simulink model "sei"  (Simulink 6.2)
settings: Solver=ode45  StartTime=0.0  StopTime=10.0  RelTol=1e-3
libraries: dsparch4 x287, cdsEpicsOut x108, cdsEpicsIn x18, cdsRms x18, Matrix8x x15, cdsSwitch1 x12, cdsProduct x9, Matrix88 x9, cdsSwitch x6, cdsSubtract8 x3, cdsRampSwitch x3, cdsSWD1 x3
(part 1 of 6)
settings Model: LastModifiedBy=rolf
settings DebuggingCC: SolverPrmCheckMsg=warning

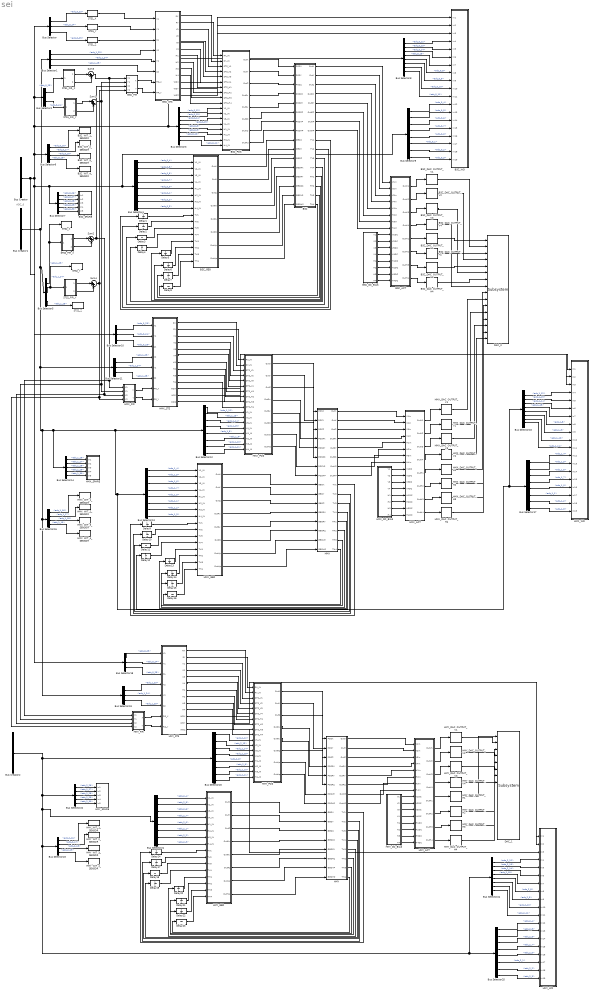
== system sei ==
  note: ADC_0
  BSC : Subsystem
  BSC_ACT : Subsystem
  BSC_DAC_OUTPUT_H{1..4} (4 alike) : cdsEpicsOut/Subsystem
  BSC_DAC_OUTPUT_V{1..4} (4 alike) : cdsEpicsOut/Subsystem
  BSC_DC_BIAS : Subsystem
  BSC_FIR : Subsystem
  BSC_GEO : Subsystem
  BSC_POS : Subsystem
  BSC_SPARE : Subsystem
  BSC_STS : Subsystem
  BSC_WD : Subsystem
  BSC_WIT_1_SENSOR : cdsEpicsOut/Subsystem
  BSC_WIT_2_SENSOR : cdsEpicsOut/Subsystem
  BSC_WIT_3_SENSOR : cdsEpicsOut/Subsystem
  BSC_WIT_4_SENSOR : cdsEpicsOut/Subsystem
  Bus Creator : BusCreator  Inputs='adc_0_0','adc_0_1','adc_0_2','adc_0_3','adc_0_4','adc_0_5','adc_0_6','adc_0_7','adc_0_8','adc_0_9','adc_0_10','adc_0_11','adc_0_12','adc_0_13','adc_0_14','adc_0_15','adc_0_16','adc_0_17','adc_0_18','adc_0_19','adc_0_20','adc_0_21','adc_0_22','adc_0_23','adc_0_24','adc_0_25','adc_0_26','adc_0_27','adc_0_28','adc_0_29','adc_0_30','adc_0_31'
  Bus Creator1 : BusCreator  Inputs='adc_1_0','adc_1_1','adc_1_2','adc_1_3','adc_1_4','adc_1_5','adc_1_6','adc_1_7','adc_1_8','adc_1_9','adc_1_10','adc_1_11','adc_1_12','adc_1_13','adc_1_14','adc_1_15','adc_1_16','adc_1_17','adc_1_18','adc_1_19','adc_1_20','adc_1_21','adc_1_22','adc_1_23','adc_1_24','adc_1_25','adc_1_26','adc_1_27','adc_1_28','adc_1_29','adc_1_30','adc_1_31'
  Bus Creator2 : BusCreator  Inputs='adc_2_0','adc_2_1','adc_2_2','adc_2_3','adc_2_4','adc_2_5','adc_2_6','adc_2_7','adc_2_8','adc_2_9','adc_2_10','adc_2_11','adc_2_12','adc_2_13','adc_2_14','adc_2_15','adc_2_16','adc_2_17','adc_2_18','adc_2_19','adc_2_20','adc_2_21','adc_2_22','adc_2_23','adc_2_24','adc_2_25','adc_2_26','adc_2_27','adc_2_28','adc_2_29','adc_2_30','adc_2_31'
  Bus Selector : BusSelector  OutputSignals=adc_0_23,adc_0_24,adc_0_25
  Bus Selector{1,5,11,19} (4 alike) : BusSelector  OutputSignals=adc_1_23,adc_1_24,adc_1_25
  Bus Selector10 : BusSelector  OutputSignals=adc_0_23,adc_0_24,adc_0_25
  Bus Selector12 : BusSelector  OutputSignals=adc_1_12,adc_1_13,adc_1_14,adc_1_15,adc_1_8,adc_1_9,adc_1_10,adc_1_11
  Bus Selector13 : BusSelector  OutputSignals=adc_1_4,adc_1_5,adc_1_6,adc_1_7,adc_1_0,adc_1_1,adc_1_2,adc_1_3
  Bus Selector14 : BusSelector  OutputSignals=adc_1_26,adc_1_27,adc_1_28,adc_1_29,adc_1_30
  Bus Selector15 : BusSelector  OutputSignals=adc_1_16,adc_1_17,adc_1_18,adc_1_19
  Bus Selector16 : BusSelector  OutputSignals=adc_1_12,adc_1_13,adc_1_14,adc_1_15,adc_1_8,adc_1_9,adc_1_10,adc_1_11
  Bus Selector17 : BusSelector  OutputSignals=adc_1_4,adc_1_5,adc_1_6,adc_1_7,adc_1_0,adc_1_1,adc_1_2,adc_1_3
  Bus Selector18 : BusSelector  OutputSignals=adc_0_23,adc_0_24,adc_0_25
  Bus Selector2 : BusSelector  OutputSignals=adc_0_23,adc_0_24
  Bus Selector20 : BusSelector  OutputSignals=adc_2_12,adc_2_13,adc_2_14,adc_2_15,adc_2_8,adc_2_9,adc_2_10,adc_2_11
  Bus Selector21 : BusSelector  OutputSignals=adc_2_4,adc_2_5,adc_2_6,adc_2_7,adc_2_0,adc_2_1,adc_2_2,adc_2_3
  Bus Selector22 : BusSelector  OutputSignals=adc_2_26,adc_2_27,adc_2_28,adc_2_29,adc_2_30
  Bus Selector23 : BusSelector  OutputSignals=adc_2_16,adc_2_17,adc_2_18,adc_2_19
  Bus Selector24 : BusSelector  OutputSignals=adc_2_12,adc_2_13,adc_2_14,adc_2_15,adc_2_8,adc_2_9,adc_2_10,adc_2_11
  Bus Selector25 : BusSelector  OutputSignals=adc_2_4,adc_2_5,adc_2_6,adc_2_7,adc_2_0,adc_2_1,adc_2_2,adc_2_3
  Bus Selector3 : BusSelector  OutputSignals=adc_0_12,adc_0_13,adc_0_14,adc_0_15,adc_0_8,adc_0_9,adc_0_10,adc_0_11
  Bus Selector4 : BusSelector  OutputSignals=adc_0_4,adc_0_5,adc_0_6,adc_0_7,adc_0_0,adc_0_1,adc_0_2,adc_0_3
  Bus Selector6 : BusSelector  OutputSignals=adc_0_16,adc_0_17,adc_0_18,adc_0_19
  Bus Selector7 : BusSelector  OutputSignals=adc_0_26,adc_0_27,adc_0_28,adc_0_29,adc_0_30
  Bus Selector8 : BusSelector  OutputSignals=adc_0_12,adc_0_13,adc_0_14,adc_0_15,adc_0_8,adc_0_9,adc_0_10,adc_0_11
  Bus Selector9 : BusSelector  OutputSignals=adc_0_4,adc_0_5,adc_0_6,adc_0_7,adc_0_0,adc_0_1,adc_0_2,adc_0_3
  DAC_0 : dac/Subsystem
  DAC_1 : dac/Subsystem
  Delay{1..24} (24 alike) : UnitDelay
  HMX : Subsystem
  HMX_ACT : Subsystem
  HMX_DAC_OUTPUT_H{1..4} (4 alike) : cdsEpicsOut/Subsystem
  HMX_DAC_OUTPUT_V{1..4} (4 alike) : cdsEpicsOut/Subsystem
  HMX_DC_BIAS : Subsystem
  HMX_FIR : Subsystem
  HMX_GEO : Subsystem
  HMX_POS : Subsystem
  HMX_SPARE : Subsystem
  HMX_STS : Subsystem
  HMX_WD : Subsystem
  HMX_WIT_1_SENSOR : cdsEpicsOut/Subsystem
  HMX_WIT_2_SENSOR : cdsEpicsOut/Subsystem
  HMX_WIT_3_SENSOR : cdsEpicsOut/Subsystem
  HMX_WIT_4_SENSOR : cdsEpicsOut/Subsystem
  HMY : Subsystem
  HMY_ACT : Subsystem
  HMY_DAC_OUTPUT_H{1..4} (4 alike) : cdsEpicsOut/Subsystem
  HMY_DAC_OUTPUT_V{1..4} (4 alike) : cdsEpicsOut/Subsystem
  HMY_DC_BIAS : Subsystem
  HMY_FIR : Subsystem
  HMY_GEO : Subsystem
  HMY_POS : Subsystem
  HMY_SPARE : Subsystem
  HMY_STS : Subsystem
  HMY_WD : Subsystem
  HMY_WIT_1_SENSOR : cdsEpicsOut/Subsystem
  HMY_WIT_2_SENSOR : cdsEpicsOut/Subsystem
  HMY_WIT_3_SENSOR : cdsEpicsOut/Subsystem
  HMY_WIT_4_SENSOR : cdsEpicsOut/Subsystem
  STS1_FIR_X : Subsystem
  STS1_FIR_Y : Subsystem
  STS1_X : cdsEpicsOut/Subsystem
  STS1_Y : cdsEpicsOut/Subsystem
  STS1_Z : cdsEpicsOut/Subsystem
  STS2_FIR_X : Subsystem
  STS2_FIR_Y : Subsystem
  STS2_X : cdsEpicsOut/Subsystem
  STS2_Y : cdsEpicsOut/Subsystem
  STS2_Z : cdsEpicsOut/Subsystem
  Sum{1..4} (4 alike) : Sum  Inputs=|++
  wires:
  BSC_FIR/1(X) -> BSC_STS/7(FIR_X)
  BSC_FIR/2(Y) -> BSC_STS/8(FIR_Y)
  BSC/1(OutX) -> BSC_ACT/1(V1In)
  BSC/2(OutY) -> BSC_ACT/2(V2In)
  BSC/3(OutZ) -> BSC_ACT/3(V3In)
  BSC/4(OutRX) -> BSC_ACT/4(V4In)
  BSC/5(OutRY) -> BSC_ACT/5(H1In)
  BSC/6(OutRZ) -> BSC_ACT/6(H2In)
  BSC/7(OutVP) -> BSC_ACT/7(H3In)
  BSC/8(OutHP) -> BSC_ACT/8(H4In)
  BSC_STS/10(H4) -> BSC_POS/10(STS_H4)
  BSC_STS/9(H3) -> BSC_POS/9(STS_H3)
  BSC_STS/8(H2) -> BSC_POS/8(STS_H2)
  BSC_STS/7(H1) -> BSC_POS/7(STS_H1)
  BSC_STS/6(V4) -> BSC_POS/6(STS_V4)
  BSC_STS/5(V3) -> BSC_POS/5(STS_V3)
  BSC_STS/4(V2) -> BSC_POS/4(STS_V2)
  BSC_STS/3(V1) -> BSC_POS/3(STS_V1)
  BSC_POS/1(OutX) -> BSC/1(POSX)
  BSC_POS/2(OutY) -> BSC/2(POSY)
  BSC_POS/3(OutZ) -> BSC/3(POSZ)
  BSC_POS/4(OutRx) -> BSC/4(POSRX)
  BSC_POS/5(OutRy) -> BSC/5(POSRY)
  BSC_POS/6(OutRZ) -> BSC/6(POSRZ)
  BSC_POS/7(OutVp) -> BSC/7(POSVP)
  BSC_POS/8(OutHp) -> BSC/8(POSHP)
  BSC_GEO/1(OutX) -> BSC/9(GEOX)
  BSC_GEO/2(OutY) -> BSC/10(GEOY)
  BSC_GEO/3(OutZ) -> BSC/11(GEOZ)
  BSC_GEO/4(OutRx) -> BSC/12(GEORX)
  BSC_GEO/5(OutRy) -> BSC/13(GEORY)
  BSC_GEO/6(OutRz) -> BSC/14(GEORZ)
  BSC_GEO/7(OutVp) -> BSC/15(GEOVP)
  BSC_GEO/8(OutHp) -> BSC/16(GEOHP)
  Bus Creator/1 -> Bus Selector/1, Bus Selector2/1, Bus Selector3/1, Bus Selector8/1, Bus Selector6/1, Bus Selector7/1, Bus Selector4/1, Bus Selector9/1, Bus Selector10/1, Bus Selector18/1
  Bus Creator1/1 -> Bus Selector1/1, Bus Selector5/1, Bus Selector11/1, Bus Selector12/1, Bus Selector13/1, Bus Selector17/1, Bus Selector16/1, Bus Selector14/1, Bus Selector15/1, Bus Selector19/1
  Bus Selector1/1 -> BSC_STS/4(X2)  "<adc_1_23>"
  Bus Selector1/2 -> BSC_STS/5(Y2)  "<adc_1_24>"
  Bus Selector1/3 -> BSC_STS/6(Z2)  "<adc_1_25>"
  Bus Selector3/1 -> BSC_POS/11(V1_IN)  "<adc_0_12>"
  Bus Selector3/2 -> BSC_POS/12(V2_IN)  "<adc_0_13>"
  Bus Selector3/3 -> BSC_POS/13(V3_IN)  "<adc_0_14>"
  Bus Selector3/4 -> BSC_POS/14(V4_IN)  "<adc_0_15>"
  Bus Selector3/5 -> BSC_POS/15(H1_IN)  "<adc_0_8>"
  Bus Selector3/6 -> BSC_POS/16(H2_IN)  "<adc_0_9>"
  Bus Selector3/7 -> BSC_POS/17(H3_IN)  "<adc_0_10>"
  Bus Selector3/8 -> BSC_POS/18(H4_IN)  "<adc_0_11>"
  Bus Selector/1 -> STS1_X/1  "<adc_0_23>"
  Bus Selector/2 -> STS1_Y/1  "<adc_0_24>"
  Bus Selector/3 -> STS1_Z/1  "<adc_0_25>"
  STS1_X/1 -> BSC_STS/1(X1)
  STS1_Y/1 -> BSC_STS/2(Y1)
  STS1_Z/1 -> BSC_STS/3(Z1)
  BSC_ACT/1(OutV1) -> BSC_DAC_OUTPUT_V1/1
  BSC_ACT/2(OutV2) -> BSC_DAC_OUTPUT_V2/1
  BSC_ACT/3(OutV3) -> BSC_DAC_OUTPUT_V3/1
  BSC_ACT/4(OutV4) -> BSC_DAC_OUTPUT_V4/1
  BSC_ACT/5(OutH1) -> BSC_DAC_OUTPUT_H1/1
  BSC_ACT/6(OutH2) -> BSC_DAC_OUTPUT_H2/1
  BSC_ACT/7(OutH3) -> BSC_DAC_OUTPUT_H3/1
  BSC_ACT/8(OutH4) -> BSC_DAC_OUTPUT_H4/1
  BSC_DC_BIAS/1(V1) -> BSC_ACT/9(V1DC)
  BSC_DC_BIAS/2(V2) -> BSC_ACT/10(V2DC)
  BSC_DC_BIAS/3(V3) -> BSC_ACT/11(V3DC)
  BSC_DC_BIAS/4(V4) -> BSC_ACT/12(V4DC)
  BSC_DC_BIAS/5(H1) -> BSC_ACT/13(H1DC)
  BSC_DC_BIAS/6(H2) -> BSC_ACT/14(H2DC)
  BSC_DC_BIAS/7(H3) -> BSC_ACT/15(H3DC)
  BSC_DC_BIAS/8(H4) -> BSC_ACT/16(H4DC)
  Delay1/1 -> BSC_GEO/9(TV1)
  Delay2/1 -> BSC_GEO/10(TV2)
  Delay8/1 -> BSC_GEO/16(TH4)
  Delay7/1 -> BSC_GEO/15(TH3)
  Delay6/1 -> BSC_GEO/14(TH2)
  Delay5/1 -> BSC_GEO/13(TH1)
  BSC/16(TH4) -> Delay8/1
  BSC/15(TH3) -> Delay7/1
  BSC/14(TH2) -> Delay6/1
  BSC/13(TH1) -> Delay5/1
  Delay3/1 -> BSC_GEO/11(TV3)
  Delay4/1 -> BSC_GEO/12(TV4)
  BSC/12(TV4) -> Delay4/1
  BSC/11(TV3) -> Delay3/1
  BSC/10(TV2) -> Delay2/1
  BSC/9(TV1) -> Delay1/1
  BSC_DAC_OUTPUT_H1/1 -> DAC_0/1
  BSC_DAC_OUTPUT_V1/1 -> DAC_0/2
  BSC_DAC_OUTPUT_H2/1 -> DAC_0/3
  BSC_DAC_OUTPUT_V2/1 -> DAC_0/4
  BSC_DAC_OUTPUT_H3/1 -> DAC_0/5
  BSC_DAC_OUTPUT_V3/1 -> DAC_0/6
  BSC_DAC_OUTPUT_V4/1 -> DAC_0/8
  Bus Selector6/1 -> BSC_WIT_1_SENSOR/1  "<adc_0_16>"
  Bus Selector6/2 -> BSC_WIT_2_SENSOR/1  "<adc_0_17>"
  Bus Selector6/3 -> BSC_WIT_3_SENSOR/1  "<adc_0_18>"
  Bus Selector6/4 -> BSC_WIT_4_SENSOR/1  "<adc_0_19>"
  Bus Selector7/1 -> BSC_SPARE/1(In1)  "<adc_0_26>"
  Bus Selector7/2 -> BSC_SPARE/2(In2)  "<adc_0_27>"
  Bus Selector7/3 -> BSC_SPARE/3(In3)  "<adc_0_28>"
  Bus Selector7/4 -> BSC_SPARE/4(In4)  "<adc_0_29>"
  Bus Selector7/5 -> BSC_SPARE/5(In5)  "<adc_0_30>"
  Bus Selector4/8 -> BSC_GEO/8(H4_IN)  "<adc_0_3>"
  Bus Selector4/7 -> BSC_GEO/7(H3_IN)  "<adc_0_2>"
  Bus Selector4/6 -> BSC_GEO/6(H2_IN)  "<adc_0_1>"
  Bus Selector4/5 -> BSC_GEO/5(H1_IN)  "<adc_0_0>"
  Bus Selector4/4 -> BSC_GEO/4(V4_IN)  "<adc_0_7>"
  Bus Selector4/3 -> BSC_GEO/3(V3_IN)  "<adc_0_6>"
  Bus Selector4/2 -> BSC_GEO/2(V2_IN)  "<adc_0_5>"
  Bus Selector4/1 -> BSC_GEO/1(V1_IN)  "<adc_0_4>"
  BSC_STS/11(WDX) -> BSC_WD/1(In1)
  BSC_STS/12(WDY) -> BSC_WD/2(In2)
  BSC_STS/13(WDZ) -> BSC_WD/3(In3)
  Bus Selector8/1 -> BSC_WD/4(In4)  "<adc_0_12>"
  Bus Selector8/2 -> BSC_WD/5(In5)  "<adc_0_13>"
  Bus Selector8/3 -> BSC_WD/6(In6)  "<adc_0_14>"
  Bus Selector8/4 -> BSC_WD/7(In7)  "<adc_0_15>"
  Bus Selector8/5 -> BSC_WD/8(In8)  "<adc_0_8>"
  Bus Selector8/6 -> BSC_WD/9(In9)  "<adc_0_9>"
  Bus Selector8/7 -> BSC_WD/10(In10)  "<adc_0_10>"
  Bus Selector8/8 -> BSC_WD/11(In11)  "<adc_0_11>"
  Bus Selector9/1 -> BSC_WD/12(In12)  "<adc_0_4>"
  Bus Selector9/2 -> BSC_WD/13(In13)  "<adc_0_5>"
  Bus Selector9/3 -> BSC_WD/14(In14)  "<adc_0_6>"
  Bus Selector9/4 -> BSC_WD/15(In15)  "<adc_0_7>"
  Bus Selector9/5 -> BSC_WD/16(In16)  "<adc_0_0>"
  Bus Selector9/6 -> BSC_WD/17(In17)  "<adc_0_1>"
  Bus Selector9/7 -> BSC_WD/18(In18)  "<adc_0_2>"
  Bus Selector9/8 -> BSC_WD/19(In19)  "<adc_0_3>"
  BSC_STS/2(RY) -> BSC_POS/1(RX_IN)
  BSC_STS/1(RX) -> BSC_POS/2(RY_IN)
  BSC_DAC_OUTPUT_H4/1 -> DAC_0/7
  Sum3/1 -> BSC_FIR/1(X1), HMX_FIR/1(X1), HMY_FIR/1(X1)
  Sum1/1 -> BSC_FIR/2(Y1), HMX_FIR/2(Y1), HMY_FIR/2(Y1)
  Bus Selector10/1 -> HMX_STS/1(X1)  "<adc_0_23>"
  Bus Selector10/2 -> HMX_STS/2(Y1)  "<adc_0_24>"
  Bus Selector10/3 -> HMX_STS/3(Z1)  "<adc_0_25>"
  Bus Selector11/1 -> HMX_STS/4(X2)  "<adc_1_23>"
  Bus Selector11/2 -> HMX_STS/5(Y2)  "<adc_1_24>"
  Bus Selector11/3 -> HMX_STS/6(Z2)  "<adc_1_25>"
  Bus Selector12/1 -> HMX_POS/11(V1_IN)  "<adc_1_12>"
  Bus Selector12/2 -> HMX_POS/12(V2_IN)  "<adc_1_13>"
  Bus Selector12/3 -> HMX_POS/13(V3_IN)  "<adc_1_14>"
  Bus Selector12/4 -> HMX_POS/14(V4_IN)  "<adc_1_15>"
  HMX_STS/10(H4) -> HMX_POS/10(STS_H4)
  HMX_STS/9(H3) -> HMX_POS/9(STS_H3)
  HMX_STS/8(H2) -> HMX_POS/8(STS_H2)
  HMX_STS/7(H1) -> HMX_POS/7(STS_H1)
  HMX_STS/6(V4) -> HMX_POS/6(STS_V4)
  HMX_STS/5(V3) -> HMX_POS/5(STS_V3)
  HMX_STS/4(V2) -> HMX_POS/4(STS_V2)
  HMX_STS/3(V1) -> HMX_POS/3(STS_V1)
  HMX_STS/1(RX) -> HMX_POS/2(RY_IN)
  HMX_STS/2(RY) -> HMX_POS/1(RX_IN)
  Bus Selector13/1 -> HMX_GEO/1(V1_IN)  "<adc_1_4>"
  Bus Selector13/2 -> HMX_GEO/2(V2_IN)  "<adc_1_5>"
  Bus Selector13/3 -> HMX_GEO/3(V3_IN)  "<adc_1_6>"
  Bus Selector13/4 -> HMX_GEO/4(V4_IN)  "<adc_1_7>"
  Bus Selector13/5 -> HMX_GEO/5(H1_IN)  "<adc_1_0>"
  Bus Selector13/6 -> HMX_GEO/6(H2_IN)  "<adc_1_1>"
  Bus Selector13/7 -> HMX_GEO/7(H3_IN)  "<adc_1_2>"
  Bus Selector13/8 -> HMX_GEO/8(H4_IN)  "<adc_1_3>"
  HMX_POS/8(OutHp) -> HMX/8(POSHP)
  HMX_POS/7(OutVp) -> HMX/7(POSVP)
  HMX_POS/6(OutRZ) -> HMX/6(POSRZ)
  HMX_POS/5(OutRy) -> HMX/5(POSRY)
  HMX_POS/4(OutRx) -> HMX/4(POSRX)
  HMX_POS/3(OutZ) -> HMX/3(POSZ)
  HMX_POS/2(OutY) -> HMX/2(POSY)
  HMX_POS/1(OutX) -> HMX/1(POSX)
  HMX_GEO/1(OutX) -> HMX/9(GEOX)
  HMX_GEO/2(OutY) -> HMX/10(GEOY)
  HMX_GEO/3(OutZ) -> HMX/11(GEOZ)
  HMX_GEO/4(OutRx) -> HMX/12(GEORX)
  HMX_GEO/5(OutRy) -> HMX/13(GEORY)
  HMX_GEO/6(OutRz) -> HMX/14(GEORZ)
  HMX_GEO/7(OutVp) -> HMX/15(GEOVP)
  HMX_GEO/8(OutHp) -> HMX/16(GEOHP)
  HMX/1(OutX) -> HMX_ACT/1(V1In)
  HMX/2(OutY) -> HMX_ACT/2(V2In)
  HMX/3(OutZ) -> HMX_ACT/3(V3In)
  HMX/4(OutRX) -> HMX_ACT/4(V4In)
  HMX/5(OutRY) -> HMX_ACT/5(H1In)
  HMX/6(OutRZ) -> HMX_ACT/6(H2In)
  HMX/7(OutVP) -> HMX_ACT/7(H3In)
  HMX/8(OutHP) -> HMX_ACT/8(H4In)
  HMX_ACT/1(OutV1) -> HMX_DAC_OUTPUT_V1/1
  HMX_ACT/2(OutV2) -> HMX_DAC_OUTPUT_V2/1
  HMX_ACT/3(OutV3) -> HMX_DAC_OUTPUT_V3/1
  HMX_ACT/4(OutV4) -> HMX_DAC_OUTPUT_V4/1
  HMX_ACT/5(OutH1) -> HMX_DAC_OUTPUT_H1/1
  HMX_ACT/6(OutH2) -> HMX_DAC_OUTPUT_H2/1
  HMX_ACT/7(OutH3) -> HMX_DAC_OUTPUT_H3/1
  HMX_ACT/8(OutH4) -> HMX_DAC_OUTPUT_H4/1
  HMX_DC_BIAS/1(V1) -> HMX_ACT/9(V1DC)
  HMX_DC_BIAS/2(V2) -> HMX_ACT/10(V2DC)
  HMX_DC_BIAS/3(V3) -> HMX_ACT/11(V3DC)
  HMX_DC_BIAS/4(V4) -> HMX_ACT/12(V4DC)
  HMX_DC_BIAS/5(H1) -> HMX_ACT/13(H1DC)
  HMX_DC_BIAS/6(H2) -> HMX_ACT/14(H2DC)
  HMX_DC_BIAS/7(H3) -> HMX_ACT/15(H3DC)
  HMX_DC_BIAS/8(H4) -> HMX_ACT/16(H4DC)
  HMX_DAC_OUTPUT_V1/1 -> DAC_0/10
  HMX_DAC_OUTPUT_H1/1 -> DAC_0/9
  HMX_DAC_OUTPUT_H2/1 -> DAC_0/11
  HMX_DAC_OUTPUT_H3/1 -> DAC_0/13
  HMX_DAC_OUTPUT_H4/1 -> DAC_0/15
  HMX_DAC_OUTPUT_V2/1 -> DAC_0/12
  HMX_DAC_OUTPUT_V3/1 -> DAC_0/14
  HMX_DAC_OUTPUT_V4/1 -> DAC_0/16
  Delay9/1 -> HMX_GEO/9(TV1)
  Delay10/1 -> HMX_GEO/10(TV2)
  Delay16/1 -> HMX_GEO/16(TH4)
  Delay15/1 -> HMX_GEO/15(TH3)
  Delay14/1 -> HMX_GEO/14(TH2)
  Delay13/1 -> HMX_GEO/13(TH1)
  HMX/16(TH4) -> Delay16/1
  HMX/15(TH3) -> Delay15/1
  HMX/14(TH2) -> Delay14/1
  HMX/13(TH1) -> Delay13/1
  Delay11/1 -> HMX_GEO/11(TV3)
  Delay12/1 -> HMX_GEO/12(TV4)
  HMX/12(TV4) -> Delay12/1
  HMX/11(TV3) -> Delay11/1
  HMX/10(TV2) -> Delay10/1
  HMX/9(TV1) -> Delay9/1
  Bus Selector14/1 -> HMX_SPARE/1(In1)  "<adc_1_26>"
  Bus Selector14/2 -> HMX_SPARE/2(In2)  "<adc_1_27>"
  Bus Selector14/3 -> HMX_SPARE/3(In3)  "<adc_1_28>"
  Bus Selector14/4 -> HMX_SPARE/4(In4)  "<adc_1_29>"
  Bus Selector14/5 -> HMX_SPARE/5(In5)  "<adc_1_30>"
  Bus Selector15/1 -> HMX_WIT_1_SENSOR/1  "<adc_1_16>"
  Bus Selector15/2 -> HMX_WIT_2_SENSOR/1  "<adc_1_17>"
  Bus Selector15/3 -> HMX_WIT_3_SENSOR/1  "<adc_1_18>"
  Bus Selector15/4 -> HMX_WIT_4_SENSOR/1  "<adc_1_19>"
  HMX_FIR/1(X) -> HMX_STS/7(FIR_X)
  HMX_FIR/2(Y) -> HMX_STS/8(FIR_Y)
  Sum4/1 -> BSC_FIR/4(Y2), HMX_FIR/4(Y2), HMY_FIR/4(Y2)
  Bus Selector5/1 -> STS2_X/1, STS2_FIR_X/1(In1)  "<adc_1_23>"
  Bus Selector5/2 -> STS2_Y/1, STS2_FIR_Y/1(In1)  "<adc_1_24>"
  Bus Selector5/3 -> STS2_Z/1  "<adc_1_25>"
  Sum2/1 -> BSC_FIR/3(X2), HMX_FIR/3(X2), HMY_FIR/3(X2)
  Bus Selector2/2 -> STS1_FIR_Y/1(In1)  "<adc_0_24>"
  Bus Selector2/1 -> STS1_FIR_X/1(In1)  "<adc_0_23>"
  STS1_FIR_Y/1(Out1) -> Sum1/1
  STS1_FIR_Y/2(Out2) -> Sum1/2
  STS1_FIR_X/1(Out1) -> Sum3/1
  STS1_FIR_X/2(Out2) -> Sum3/2
  STS2_FIR_Y/1(Out1) -> Sum4/1
  STS2_FIR_Y/2(Out2) -> Sum4/2
  STS2_FIR_X/1(Out1) -> Sum2/1
  STS2_FIR_X/2(Out2) -> Sum2/2
  Bus Selector16/1 -> HMX_WD/4(In4)  "<adc_1_12>"
  Bus Selector16/2 -> HMX_WD/5(In5)  "<adc_1_13>"
  Bus Selector16/3 -> HMX_WD/6(In6)  "<adc_1_14>"
  Bus Selector16/4 -> HMX_WD/7(In7)  "<adc_1_15>"
  Bus Selector16/5 -> HMX_WD/8(In8)  "<adc_1_8>"
  Bus Selector16/6 -> HMX_WD/9(In9)  "<adc_1_9>"
  Bus Selector16/7 -> HMX_WD/10(In10)  "<adc_1_10>"
  Bus Selector16/8 -> HMX_WD/11(In11)  "<adc_1_11>"
  Bus Selector17/1 -> HMX_WD/12(In12)  "<adc_1_4>"
  Bus Selector17/2 -> HMX_WD/13(In13)  "<adc_1_5>"
  Bus Selector17/3 -> HMX_WD/14(In14)  "<adc_1_6>"
  Bus Selector17/4 -> HMX_WD/15(In15)  "<adc_1_7>"
  Bus Selector17/5 -> HMX_WD/16(In16)  "<adc_1_0>"
  Bus Selector17/6 -> HMX_WD/17(In17)  "<adc_1_1>"
  Bus Selector17/7 -> HMX_WD/18(In18)  "<adc_1_2>"
  Bus Selector17/8 -> HMX_WD/19(In19)  "<adc_1_3>"
  HMX_STS/11(WDX) -> HMX_WD/1(In1)
  HMX_STS/12(WDY) -> HMX_WD/2(In2)
  HMX_STS/13(WDZ) -> HMX_WD/3(In3)
  Bus Selector18/1 -> HMY_STS/1(X1)  "<adc_0_23>"
  Bus Selector18/2 -> HMY_STS/2(Y1)  "<adc_0_24>"
  Bus Selector18/3 -> HMY_STS/3(Z1)  "<adc_0_25>"
  Bus Selector19/1 -> HMY_STS/4(X2)  "<adc_1_23>"
  Bus Selector19/2 -> HMY_STS/5(Y2)  "<adc_1_24>"
  Bus Selector19/3 -> HMY_STS/6(Z2)  "<adc_1_25>"
  Bus Selector20/1 -> HMY_POS/11(V1_IN)  "<adc_2_12>"
  Bus Selector20/2 -> HMY_POS/12(V2_IN)  "<adc_2_13>"
  Bus Selector20/3 -> HMY_POS/13(V3_IN)  "<adc_2_14>"
  Bus Selector20/4 -> HMY_POS/14(V4_IN)  "<adc_2_15>"
  Bus Selector20/5 -> HMY_POS/15(H1_IN)  "<adc_2_8>"
  Bus Selector20/6 -> HMY_POS/16(H2_IN)  "<adc_2_9>"
  Bus Selector20/7 -> HMY_POS/17(H3_IN)  "<adc_2_10>"
  Bus Selector20/8 -> HMY_POS/18(H4_IN)  "<adc_2_11>"
  HMY_STS/10(H4) -> HMY_POS/10(STS_H4)
  HMY_STS/9(H3) -> HMY_POS/9(STS_H3)
  HMY_STS/8(H2) -> HMY_POS/8(STS_H2)
  HMY_STS/7(H1) -> HMY_POS/7(STS_H1)
  HMY_STS/6(V4) -> HMY_POS/6(STS_V4)
  HMY_STS/5(V3) -> HMY_POS/5(STS_V3)
  HMY_STS/4(V2) -> HMY_POS/4(STS_V2)
  HMY_STS/3(V1) -> HMY_POS/3(STS_V1)
  HMY_STS/1(RX) -> HMY_POS/2(RY_IN)
  HMY_STS/2(RY) -> HMY_POS/1(RX_IN)
  Bus Selector21/1 -> HMY_GEO/1(V1_IN)  "<adc_2_4>"
  Bus Selector21/2 -> HMY_GEO/2(V2_IN)  "<adc_2_5>"
  Bus Selector21/3 -> HMY_GEO/3(V3_IN)  "<adc_2_6>"
  Bus Selector21/4 -> HMY_GEO/4(V4_IN)  "<adc_2_7>"
  Bus Selector21/5 -> HMY_GEO/5(H1_IN)  "<adc_2_0>"
  Bus Selector21/6 -> HMY_GEO/6(H2_IN)  "<adc_2_1>"
  Bus Selector21/7 -> HMY_GEO/7(H3_IN)  "<adc_2_2>"
  Bus Selector21/8 -> HMY_GEO/8(H4_IN)  "<adc_2_3>"
  HMY_POS/8(OutHp) -> HMY/8(POSHP)
  HMY_POS/7(OutVp) -> HMY/7(POSVP)
  HMY_POS/6(OutRZ) -> HMY/6(POSRZ)
  HMY_POS/5(OutRy) -> HMY/5(POSRY)
  HMY_POS/4(OutRx) -> HMY/4(POSRX)
  HMY_POS/3(OutZ) -> HMY/3(POSZ)
  HMY_POS/2(OutY) -> HMY/2(POSY)
  HMY_POS/1(OutX) -> HMY/1(POSX)
  HMY_GEO/1(OutX) -> HMY/9(GEOX)
  HMY_GEO/2(OutY) -> HMY/10(GEOY)
  HMY_GEO/3(OutZ) -> HMY/11(GEOZ)
  HMY_GEO/4(OutRx) -> HMY/12(GEORX)
  HMY_GEO/5(OutRy) -> HMY/13(GEORY)
  HMY_GEO/6(OutRz) -> HMY/14(GEORZ)
  HMY_GEO/7(OutVp) -> HMY/15(GEOVP)
  HMY_GEO/8(OutHp) -> HMY/16(GEOHP)
  HMY/1(OutX) -> HMY_ACT/1(V1In)
  HMY/2(OutY) -> HMY_ACT/2(V2In)
  HMY/3(OutZ) -> HMY_ACT/3(V3In)
  HMY/4(OutRX) -> HMY_ACT/4(V4In)
  HMY/5(OutRY) -> HMY_ACT/5(H1In)
  HMY/6(OutRZ) -> HMY_ACT/6(H2In)
  HMY/7(OutVP) -> HMY_ACT/7(H3In)
  HMY/8(OutHP) -> HMY_ACT/8(H4In)
  HMY_ACT/1(OutV1) -> HMY_DAC_OUTPUT_V1/1
  HMY_ACT/2(OutV2) -> HMY_DAC_OUTPUT_V2/1
  HMY_ACT/3(OutV3) -> HMY_DAC_OUTPUT_V3/1
  HMY_ACT/4(OutV4) -> HMY_DAC_OUTPUT_V4/1
  HMY_ACT/5(OutH1) -> HMY_DAC_OUTPUT_H1/1
  HMY_ACT/6(OutH2) -> HMY_DAC_OUTPUT_H2/1
  HMY_ACT/7(OutH3) -> HMY_DAC_OUTPUT_H3/1
  HMY_ACT/8(OutH4) -> HMY_DAC_OUTPUT_H4/1
  HMY_DC_BIAS/1(V1) -> HMY_ACT/9(V1DC)
  HMY_DC_BIAS/2(V2) -> HMY_ACT/10(V2DC)
  HMY_DC_BIAS/3(V3) -> HMY_ACT/11(V3DC)
  HMY_DC_BIAS/4(V4) -> HMY_ACT/12(V4DC)
  HMY_DC_BIAS/5(H1) -> HMY_ACT/13(H1DC)
  HMY_DC_BIAS/6(H2) -> HMY_ACT/14(H2DC)
  HMY_DC_BIAS/7(H3) -> HMY_ACT/15(H3DC)
  HMY_DC_BIAS/8(H4) -> HMY_ACT/16(H4DC)
  Delay24/1 -> HMY_GEO/9(TV1)
  Delay17/1 -> HMY_GEO/10(TV2)
  Delay23/1 -> HMY_GEO/16(TH4)
  Delay22/1 -> HMY_GEO/15(TH3)
  Delay21/1 -> HMY_GEO/14(TH2)
  Delay20/1 -> HMY_GEO/13(TH1)
  HMY/16(TH4) -> Delay23/1
  HMY/15(TH3) -> Delay22/1
  HMY/14(TH2) -> Delay21/1
  HMY/13(TH1) -> Delay20/1
  Delay18/1 -> HMY_GEO/11(TV3)
  Delay19/1 -> HMY_GEO/12(TV4)
  HMY/12(TV4) -> Delay19/1
  HMY/11(TV3) -> Delay18/1
  HMY/10(TV2) -> Delay17/1
  HMY/9(TV1) -> Delay24/1
  Bus Selector22/1 -> HMY_SPARE/1(In1)  "<adc_2_26>"
  Bus Selector22/2 -> HMY_SPARE/2(In2)  "<adc_2_27>"
  Bus Selector22/3 -> HMY_SPARE/3(In3)  "<adc_2_28>"
  Bus Selector22/4 -> HMY_SPARE/4(In4)  "<adc_2_29>"
  Bus Selector22/5 -> HMY_SPARE/5(In5)  "<adc_2_30>"
  Bus Selector23/1 -> HMY_WIT_1_SENSOR/1  "<adc_2_16>"
  Bus Selector23/2 -> HMY_WIT_2_SENSOR/1  "<adc_2_17>"
  Bus Selector23/3 -> HMY_WIT_3_SENSOR/1  "<adc_2_18>"
  Bus Selector23/4 -> HMY_WIT_4_SENSOR/1  "<adc_2_19>"
  HMY_FIR/1(X) -> HMY_STS/7(FIR_X)
  HMY_FIR/2(Y) -> HMY_STS/8(FIR_Y)
  Bus Creator2/1 -> Bus Selector22/1, Bus Selector21/1, Bus Selector23/1, Bus Selector25/1, Bus Selector24/1, Bus Selector20/1
  Bus Selector24/1 -> HMY_WD/4(In4)  "<adc_2_12>"
  Bus Selector24/2 -> HMY_WD/5(In5)  "<adc_2_13>"
  Bus Selector24/3 -> HMY_WD/6(In6)  "<adc_2_14>"
  Bus Selector24/4 -> HMY_WD/7(In7)  "<adc_2_15>"
  Bus Selector24/5 -> HMY_WD/8(In8)  "<adc_2_8>"
  Bus Selector24/6 -> HMY_WD/9(In9)  "<adc_2_9>"
  Bus Selector24/7 -> HMY_WD/10(In10)  "<adc_2_10>"
  Bus Selector24/8 -> HMY_WD/11(In11)  "<adc_2_11>"
  Bus Selector25/1 -> HMY_WD/12(In12)  "<adc_2_4>"
  Bus Selector25/2 -> HMY_WD/13(In13)  "<adc_2_5>"
  Bus Selector25/3 -> HMY_WD/14(In14)  "<adc_2_6>"
  Bus Selector25/4 -> HMY_WD/15(In15)  "<adc_2_7>"
  Bus Selector25/5 -> HMY_WD/16(In16)  "<adc_2_0>"
  Bus Selector25/6 -> HMY_WD/17(In17)  "<adc_2_1>"
  Bus Selector25/7 -> HMY_WD/18(In18)  "<adc_2_2>"
  Bus Selector25/8 -> HMY_WD/19(In19)  "<adc_2_3>"
  HMY_STS/13(WDZ) -> HMY_WD/3(In3)
  HMY_STS/12(WDY) -> HMY_WD/2(In2)
  HMY_STS/11(WDX) -> HMY_WD/1(In1)
  HMY_DAC_OUTPUT_H1/1 -> DAC_1/1
  HMY_DAC_OUTPUT_V1/1 -> DAC_1/2
  HMY_DAC_OUTPUT_H2/1 -> DAC_1/3
  HMY_DAC_OUTPUT_V2/1 -> DAC_1/4
  HMY_DAC_OUTPUT_H3/1 -> DAC_1/5
  HMY_DAC_OUTPUT_V3/1 -> DAC_1/6
  HMY_DAC_OUTPUT_H4/1 -> DAC_1/7
  HMY_DAC_OUTPUT_V4/1 -> DAC_1/8
  Bus Selector12/5 -> HMX_POS/15(H1_IN)  "<adc_1_8>"
  Bus Selector12/6 -> HMX_POS/16(H2_IN)  "<adc_1_9>"
  Bus Selector12/7 -> HMX_POS/17(H3_IN)  "<adc_1_10>"
  Bus Selector12/8 -> HMX_POS/18(H4_IN)  "<adc_1_11>"

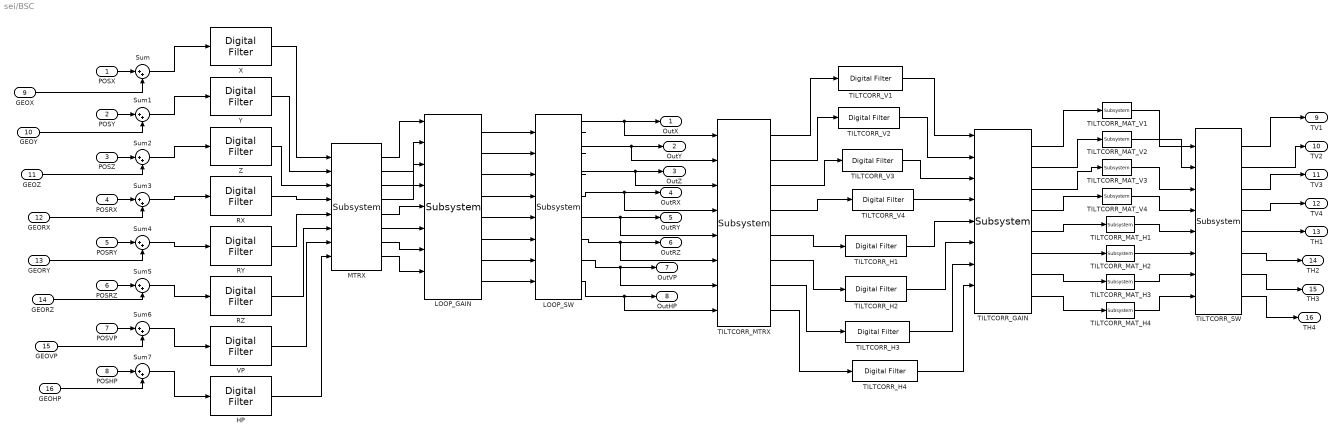
== system sei/BSC ==
  POSX : Inport  Port=1  LatchInput=off
  POSY : Inport  Port=2  LatchInput=off
  POSZ : Inport  Port=3  LatchInput=off
  POSRX : Inport  Port=4  LatchInput=off
  POSRY : Inport  Port=5  LatchInput=off
  POSRZ : Inport  Port=6  LatchInput=off
  POSVP : Inport  Port=7  LatchInput=off
  POSHP : Inport  Port=8  LatchInput=off
  GEOX : Inport  Port=9  LatchInput=off
  GEOY : Inport  Port=10  LatchInput=off
  GEOZ : Inport  Port=11  LatchInput=off
  GEORX : Inport  Port=12  LatchInput=off
  GEORY : Inport  Port=13  LatchInput=off
  GEORZ : Inport  Port=14  LatchInput=off
  GEOVP : Inport  Port=15  LatchInput=off
  GEOHP : Inport  Port=16  LatchInput=off
  HP : dsparch4/Digital Filter  DialogController=dspDDGCreate  DialogControllerArgs=DataTag0  TypePopup=IIR (poles & zeros)  IIRFiltStruct=Direct form II transposed  AllPoleFiltStruct=Direct form  FIRFiltStruct=Direct form  CoeffSource=Specify via dialog  NumCoeffs=[1 2]  DenCoeffs=[1 0.1]  BiQuadCoeffs=[1 0.3 0.4 1 0.1 0.2]  LatticeCoeffs=[0.2 0.4]  denIgnore=on  FiltPerSampPopup=One filter per frame  IC=0  ICnum=0  ICden=0  roundingMode=Floor  overflowMode=off  ScaleValues=1  scaleValueFracLength=14  stageInFracLength=15  stageOutFracLength=15
  LOOP_GAIN : cdsProduct/Subsystem
      settings: AttributesFormatString=%<ReferenceBlock>
  LOOP_SW : cdsSwitch1/Subsystem
      settings: AttributesFormatString=%<ReferenceBlock>
  MTRX : Matrix8x/Subsystem
  RX : dsparch4/Digital Filter  DialogController=dspDDGCreate  DialogControllerArgs=DataTag1  TypePopup=IIR (poles & zeros)  IIRFiltStruct=Direct form II transposed  AllPoleFiltStruct=Direct form  FIRFiltStruct=Direct form  CoeffSource=Specify via dialog  NumCoeffs=[1 2]  DenCoeffs=[1 0.1]  BiQuadCoeffs=[1 0.3 0.4 1 0.1 0.2]  LatticeCoeffs=[0.2 0.4]  denIgnore=on  FiltPerSampPopup=One filter per frame  IC=0  ICnum=0  ICden=0  roundingMode=Floor  overflowMode=off  ScaleValues=1  scaleValueFracLength=14  stageInFracLength=15  stageOutFracLength=15
  RY : dsparch4/Digital Filter  DialogController=dspDDGCreate  DialogControllerArgs=DataTag2  TypePopup=IIR (poles & zeros)  IIRFiltStruct=Direct form II transposed  AllPoleFiltStruct=Direct form  FIRFiltStruct=Direct form  CoeffSource=Specify via dialog  NumCoeffs=[1 2]  DenCoeffs=[1 0.1]  BiQuadCoeffs=[1 0.3 0.4 1 0.1 0.2]  LatticeCoeffs=[0.2 0.4]  denIgnore=on  FiltPerSampPopup=One filter per frame  IC=0  ICnum=0  ICden=0  roundingMode=Floor  overflowMode=off  ScaleValues=1  scaleValueFracLength=14  stageInFracLength=15  stageOutFracLength=15
  RZ : dsparch4/Digital Filter  DialogController=dspDDGCreate  DialogControllerArgs=DataTag3  TypePopup=IIR (poles & zeros)  IIRFiltStruct=Direct form II transposed  AllPoleFiltStruct=Direct form  FIRFiltStruct=Direct form  CoeffSource=Specify via dialog  NumCoeffs=[1 2]  DenCoeffs=[1 0.1]  BiQuadCoeffs=[1 0.3 0.4 1 0.1 0.2]  LatticeCoeffs=[0.2 0.4]  denIgnore=on  FiltPerSampPopup=One filter per frame  IC=0  ICnum=0  ICden=0  roundingMode=Floor  overflowMode=off  ScaleValues=1  scaleValueFracLength=14  stageInFracLength=15  stageOutFracLength=15
  Sum{,1..7} (8 alike) : Sum  Inputs=|++
  TILTCORR_GAIN : cdsProduct/Subsystem
      settings: AttributesFormatString=%<ReferenceBlock>
  TILTCORR_H1 : dsparch4/Digital Filter  DialogController=dspDDGCreate  DialogControllerArgs=DataTag4  TypePopup=IIR (poles & zeros)  IIRFiltStruct=Direct form II transposed  AllPoleFiltStruct=Direct form  FIRFiltStruct=Direct form  CoeffSource=Specify via dialog  NumCoeffs=[1 2]  DenCoeffs=[1 0.1]  BiQuadCoeffs=[1 0.3 0.4 1 0.1 0.2]  LatticeCoeffs=[0.2 0.4]  denIgnore=on  FiltPerSampPopup=One filter per frame  IC=0  ICnum=0  ICden=0  roundingMode=Floor  overflowMode=off  ScaleValues=1  scaleValueFracLength=14  stageInFracLength=15  stageOutFracLength=15
  TILTCORR_H2 : dsparch4/Digital Filter  DialogController=dspDDGCreate  DialogControllerArgs=DataTag5  TypePopup=IIR (poles & zeros)  IIRFiltStruct=Direct form II transposed  AllPoleFiltStruct=Direct form  FIRFiltStruct=Direct form  CoeffSource=Specify via dialog  NumCoeffs=[1 2]  DenCoeffs=[1 0.1]  BiQuadCoeffs=[1 0.3 0.4 1 0.1 0.2]  LatticeCoeffs=[0.2 0.4]  denIgnore=on  FiltPerSampPopup=One filter per frame  IC=0  ICnum=0  ICden=0  roundingMode=Floor  overflowMode=off  ScaleValues=1  scaleValueFracLength=14  stageInFracLength=15  stageOutFracLength=15
  TILTCORR_H3 : dsparch4/Digital Filter  DialogController=dspDDGCreate  DialogControllerArgs=DataTag6  TypePopup=IIR (poles & zeros)  IIRFiltStruct=Direct form II transposed  AllPoleFiltStruct=Direct form  FIRFiltStruct=Direct form  CoeffSource=Specify via dialog  NumCoeffs=[1 2]  DenCoeffs=[1 0.1]  BiQuadCoeffs=[1 0.3 0.4 1 0.1 0.2]  LatticeCoeffs=[0.2 0.4]  denIgnore=on  FiltPerSampPopup=One filter per frame  IC=0  ICnum=0  ICden=0  roundingMode=Floor  overflowMode=off  ScaleValues=1  scaleValueFracLength=14  stageInFracLength=15  stageOutFracLength=15
  TILTCORR_H4 : dsparch4/Digital Filter  DialogController=dspDDGCreate  DialogControllerArgs=DataTag7  TypePopup=IIR (poles & zeros)  IIRFiltStruct=Direct form II transposed  AllPoleFiltStruct=Direct form  FIRFiltStruct=Direct form  CoeffSource=Specify via dialog  NumCoeffs=[1 2]  DenCoeffs=[1 0.1]  BiQuadCoeffs=[1 0.3 0.4 1 0.1 0.2]  LatticeCoeffs=[0.2 0.4]  denIgnore=on  FiltPerSampPopup=One filter per frame  IC=0  ICnum=0  ICden=0  roundingMode=Floor  overflowMode=off  ScaleValues=1  scaleValueFracLength=14  stageInFracLength=15  stageOutFracLength=15
  TILTCORR_MAT_H{1..4} (4 alike) : cdsEpicsOut/Subsystem
  TILTCORR_MAT_V{1..4} (4 alike) : cdsEpicsOut/Subsystem
  TILTCORR_MTRX : Matrix8x/Subsystem
  TILTCORR_SW : cdsSwitch1/Subsystem
      settings: AttributesFormatString=%<ReferenceBlock>
  TILTCORR_V1 : dsparch4/Digital Filter  DialogController=dspDDGCreate  DialogControllerArgs=DataTag8  TypePopup=IIR (poles & zeros)  IIRFiltStruct=Direct form II transposed  AllPoleFiltStruct=Direct form  FIRFiltStruct=Direct form  CoeffSource=Specify via dialog  NumCoeffs=[1 2]  DenCoeffs=[1 0.1]  BiQuadCoeffs=[1 0.3 0.4 1 0.1 0.2]  LatticeCoeffs=[0.2 0.4]  denIgnore=on  FiltPerSampPopup=One filter per frame  IC=0  ICnum=0  ICden=0  roundingMode=Floor  overflowMode=off  ScaleValues=1  scaleValueFracLength=14  stageInFracLength=15  stageOutFracLength=15
  TILTCORR_V2 : dsparch4/Digital Filter  DialogController=dspDDGCreate  DialogControllerArgs=DataTag9  TypePopup=IIR (poles & zeros)  IIRFiltStruct=Direct form II transposed  AllPoleFiltStruct=Direct form  FIRFiltStruct=Direct form  CoeffSource=Specify via dialog  NumCoeffs=[1 2]  DenCoeffs=[1 0.1]  BiQuadCoeffs=[1 0.3 0.4 1 0.1 0.2]  LatticeCoeffs=[0.2 0.4]  denIgnore=on  FiltPerSampPopup=One filter per frame  IC=0  ICnum=0  ICden=0  roundingMode=Floor  overflowMode=off  ScaleValues=1  scaleValueFracLength=14  stageInFracLength=15  stageOutFracLength=15
  TILTCORR_V3 : dsparch4/Digital Filter  DialogController=dspDDGCreate  DialogControllerArgs=DataTag10  TypePopup=IIR (poles & zeros)  IIRFiltStruct=Direct form II transposed  AllPoleFiltStruct=Direct form  FIRFiltStruct=Direct form  CoeffSource=Specify via dialog  NumCoeffs=[1 2]  DenCoeffs=[1 0.1]  BiQuadCoeffs=[1 0.3 0.4 1 0.1 0.2]  LatticeCoeffs=[0.2 0.4]  denIgnore=on  FiltPerSampPopup=One filter per frame  IC=0  ICnum=0  ICden=0  roundingMode=Floor  overflowMode=off  ScaleValues=1  scaleValueFracLength=14  stageInFracLength=15  stageOutFracLength=15
  TILTCORR_V4 : dsparch4/Digital Filter  DialogController=dspDDGCreate  DialogControllerArgs=DataTag11  TypePopup=IIR (poles & zeros)  IIRFiltStruct=Direct form II transposed  AllPoleFiltStruct=Direct form  FIRFiltStruct=Direct form  CoeffSource=Specify via dialog  NumCoeffs=[1 2]  DenCoeffs=[1 0.1]  BiQuadCoeffs=[1 0.3 0.4 1 0.1 0.2]  LatticeCoeffs=[0.2 0.4]  denIgnore=on  FiltPerSampPopup=One filter per frame  IC=0  ICnum=0  ICden=0  roundingMode=Floor  overflowMode=off  ScaleValues=1  scaleValueFracLength=14  stageInFracLength=15  stageOutFracLength=15
  VP : dsparch4/Digital Filter  DialogController=dspDDGCreate  DialogControllerArgs=DataTag12  TypePopup=IIR (poles & zeros)  IIRFiltStruct=Direct form II transposed  AllPoleFiltStruct=Direct form  FIRFiltStruct=Direct form  CoeffSource=Specify via dialog  NumCoeffs=[1 2]  DenCoeffs=[1 0.1]  BiQuadCoeffs=[1 0.3 0.4 1 0.1 0.2]  LatticeCoeffs=[0.2 0.4]  denIgnore=on  FiltPerSampPopup=One filter per frame  IC=0  ICnum=0  ICden=0  roundingMode=Floor  overflowMode=off  ScaleValues=1  scaleValueFracLength=14  stageInFracLength=15  stageOutFracLength=15
  X : dsparch4/Digital Filter  DialogController=dspDDGCreate  DialogControllerArgs=DataTag13  TypePopup=IIR (poles & zeros)  IIRFiltStruct=Direct form II transposed  AllPoleFiltStruct=Direct form  FIRFiltStruct=Direct form  CoeffSource=Specify via dialog  NumCoeffs=[1 2]  DenCoeffs=[1 0.1]  BiQuadCoeffs=[1 0.3 0.4 1 0.1 0.2]  LatticeCoeffs=[0.2 0.4]  denIgnore=on  FiltPerSampPopup=One filter per frame  IC=0  ICnum=0  ICden=0  roundingMode=Floor  overflowMode=off  ScaleValues=1  scaleValueFracLength=14  stageInFracLength=15  stageOutFracLength=15
  Y : dsparch4/Digital Filter  DialogController=dspDDGCreate  DialogControllerArgs=DataTag14  TypePopup=IIR (poles & zeros)  IIRFiltStruct=Direct form II transposed  AllPoleFiltStruct=Direct form  FIRFiltStruct=Direct form  CoeffSource=Specify via dialog  NumCoeffs=[1 2]  DenCoeffs=[1 0.1]  BiQuadCoeffs=[1 0.3 0.4 1 0.1 0.2]  LatticeCoeffs=[0.2 0.4]  denIgnore=on  FiltPerSampPopup=One filter per frame  IC=0  ICnum=0  ICden=0  roundingMode=Floor  overflowMode=off  ScaleValues=1  scaleValueFracLength=14  stageInFracLength=15  stageOutFracLength=15
  Z : dsparch4/Digital Filter  DialogController=dspDDGCreate  DialogControllerArgs=DataTag15  TypePopup=IIR (poles & zeros)  IIRFiltStruct=Direct form II transposed  AllPoleFiltStruct=Direct form  FIRFiltStruct=Direct form  CoeffSource=Specify via dialog  NumCoeffs=[1 2]  DenCoeffs=[1 0.1]  BiQuadCoeffs=[1 0.3 0.4 1 0.1 0.2]  LatticeCoeffs=[0.2 0.4]  denIgnore=on  FiltPerSampPopup=One filter per frame  IC=0  ICnum=0  ICden=0  roundingMode=Floor  overflowMode=off  ScaleValues=1  scaleValueFracLength=14  stageInFracLength=15  stageOutFracLength=15
  OutX : Outport
  OutY : Outport  Port=2
  OutZ : Outport  Port=3
  OutRX : Outport  Port=4
  OutRY : Outport  Port=5
  OutRZ : Outport  Port=6
  OutVP : Outport  Port=7
  OutHP : Outport  Port=8
  TV1 : Outport  Port=9
  TV2 : Outport  Port=10
  TV3 : Outport  Port=11
  TV4 : Outport  Port=12
  TH1 : Outport  Port=13
  TH2 : Outport  Port=14
  TH3 : Outport  Port=15
  TH4 : Outport  Port=16
  wires:
  Sum/1 -> X/1
  Sum1/1 -> Y/1
  Sum2/1 -> Z/1
  Sum3/1 -> RX/1
  Sum4/1 -> RY/1
  Sum5/1 -> RZ/1
  Sum6/1 -> VP/1
  Sum7/1 -> HP/1
  X/1 -> MTRX/1
  Y/1 -> MTRX/2
  Z/1 -> MTRX/3
  RX/1 -> MTRX/4
  RY/1 -> MTRX/5
  RZ/1 -> MTRX/6
  VP/1 -> MTRX/7
  HP/1 -> MTRX/8
  POSX/1 -> Sum/1
  GEOX/1 -> Sum/2
  POSY/1 -> Sum1/1
  GEOY/1 -> Sum1/2
  POSZ/1 -> Sum2/1
  GEOZ/1 -> Sum2/2
  POSRX/1 -> Sum3/1
  GEORX/1 -> Sum3/2
  POSRY/1 -> Sum4/1
  GEORY/1 -> Sum4/2
  POSRZ/1 -> Sum5/1
  GEORZ/1 -> Sum5/2
  POSVP/1 -> Sum6/1
  GEOVP/1 -> Sum6/2
  POSHP/1 -> Sum7/1
  GEOHP/1 -> Sum7/2
  LOOP_GAIN/1 -> LOOP_SW/1
  LOOP_GAIN/2 -> LOOP_SW/2
  LOOP_GAIN/3 -> LOOP_SW/3
  LOOP_GAIN/4 -> LOOP_SW/4
  LOOP_GAIN/5 -> LOOP_SW/5
  LOOP_GAIN/6 -> LOOP_SW/6
  LOOP_GAIN/7 -> LOOP_SW/7
  LOOP_GAIN/8 -> LOOP_SW/8
  LOOP_SW/1 -> OutX/1, TILTCORR_MTRX/1
  LOOP_SW/2 -> OutY/1, TILTCORR_MTRX/2
  LOOP_SW/3 -> OutZ/1, TILTCORR_MTRX/3
  LOOP_SW/4 -> OutRX/1, TILTCORR_MTRX/4
  LOOP_SW/5 -> OutRY/1, TILTCORR_MTRX/5
  LOOP_SW/6 -> OutRZ/1, TILTCORR_MTRX/6
  LOOP_SW/7 -> OutVP/1, TILTCORR_MTRX/7
  LOOP_SW/8 -> OutHP/1, TILTCORR_MTRX/8
  MTRX/1 -> LOOP_GAIN/1
  MTRX/2 -> LOOP_GAIN/2
  MTRX/3 -> LOOP_GAIN/3
  MTRX/4 -> LOOP_GAIN/4
  MTRX/5 -> LOOP_GAIN/5
  MTRX/6 -> LOOP_GAIN/6
  MTRX/7 -> LOOP_GAIN/7
  MTRX/8 -> LOOP_GAIN/8
  TILTCORR_MTRX/1 -> TILTCORR_V1/1
  TILTCORR_MTRX/2 -> TILTCORR_V2/1
  TILTCORR_MTRX/3 -> TILTCORR_V3/1
  TILTCORR_MTRX/4 -> TILTCORR_V4/1
  TILTCORR_MTRX/5 -> TILTCORR_H1/1
  TILTCORR_MTRX/6 -> TILTCORR_H2/1
  TILTCORR_MTRX/7 -> TILTCORR_H3/1
  TILTCORR_MTRX/8 -> TILTCORR_H4/1
  TILTCORR_V1/1 -> TILTCORR_GAIN/1
  TILTCORR_V2/1 -> TILTCORR_GAIN/2
  TILTCORR_V3/1 -> TILTCORR_GAIN/3
  TILTCORR_V4/1 -> TILTCORR_GAIN/4
  TILTCORR_H1/1 -> TILTCORR_GAIN/5
  TILTCORR_H2/1 -> TILTCORR_GAIN/6
  TILTCORR_H3/1 -> TILTCORR_GAIN/7
  TILTCORR_H4/1 -> TILTCORR_GAIN/8
  TILTCORR_GAIN/1 -> TILTCORR_MAT_V1/1
  TILTCORR_GAIN/2 -> TILTCORR_MAT_V2/1
  TILTCORR_GAIN/3 -> TILTCORR_MAT_V3/1
  TILTCORR_GAIN/4 -> TILTCORR_MAT_V4/1
  TILTCORR_GAIN/5 -> TILTCORR_MAT_H1/1
  TILTCORR_GAIN/6 -> TILTCORR_MAT_H2/1
  TILTCORR_GAIN/7 -> TILTCORR_MAT_H3/1
  TILTCORR_GAIN/8 -> TILTCORR_MAT_H4/1
  TILTCORR_MAT_V1/1 -> TILTCORR_SW/1
  TILTCORR_MAT_V2/1 -> TILTCORR_SW/2
  TILTCORR_MAT_V3/1 -> TILTCORR_SW/3
  TILTCORR_MAT_V4/1 -> TILTCORR_SW/4
  TILTCORR_MAT_H1/1 -> TILTCORR_SW/5
  TILTCORR_MAT_H2/1 -> TILTCORR_SW/6
  TILTCORR_MAT_H3/1 -> TILTCORR_SW/7
  TILTCORR_MAT_H4/1 -> TILTCORR_SW/8
  TILTCORR_SW/1 -> TV1/1
  TILTCORR_SW/2 -> TV2/1
  TILTCORR_SW/3 -> TV3/1
  TILTCORR_SW/4 -> TV4/1
  TILTCORR_SW/5 -> TH1/1
  TILTCORR_SW/6 -> TH2/1
  TILTCORR_SW/7 -> TH3/1
  TILTCORR_SW/8 -> TH4/1

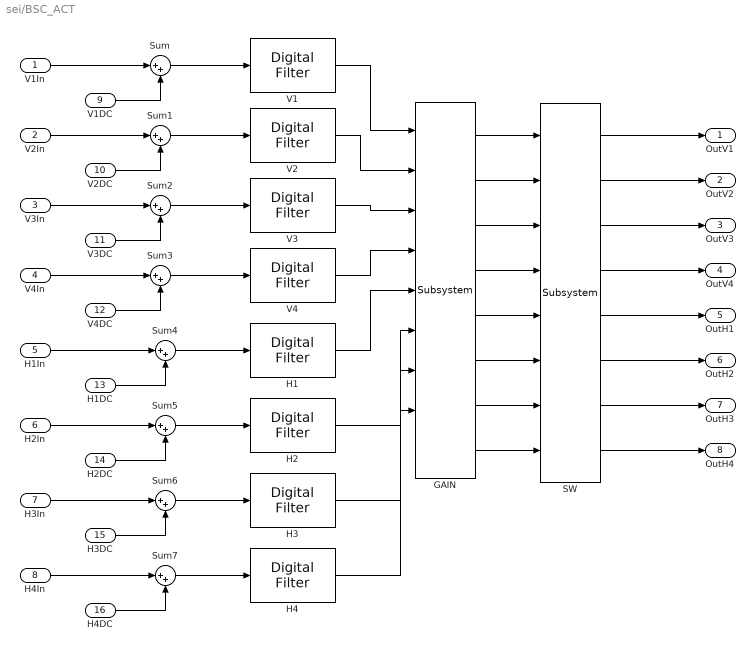
== system sei/BSC_ACT ==
  V1In : Inport  Port=1  LatchInput=off
  V2In : Inport  Port=2  LatchInput=off
  V3In : Inport  Port=3  LatchInput=off
  V4In : Inport  Port=4  LatchInput=off
  H1In : Inport  Port=5  LatchInput=off
  H2In : Inport  Port=6  LatchInput=off
  H3In : Inport  Port=7  LatchInput=off
  H4In : Inport  Port=8  LatchInput=off
  V1DC : Inport  Port=9  LatchInput=off
  V2DC : Inport  Port=10  LatchInput=off
  V3DC : Inport  Port=11  LatchInput=off
  V4DC : Inport  Port=12  LatchInput=off
  H1DC : Inport  Port=13  LatchInput=off
  H2DC : Inport  Port=14  LatchInput=off
  H3DC : Inport  Port=15  LatchInput=off
  H4DC : Inport  Port=16  LatchInput=off
  GAIN : cdsProduct/Subsystem
  H1 : dsparch4/Digital Filter  DialogController=dspDDGCreate  DialogControllerArgs=DataTag16  TypePopup=IIR (poles & zeros)  IIRFiltStruct=Direct form II transposed  AllPoleFiltStruct=Direct form  FIRFiltStruct=Direct form  CoeffSource=Specify via dialog  NumCoeffs=[1 2]  DenCoeffs=[1 0.1]  BiQuadCoeffs=[1 0.3 0.4 1 0.1 0.2]  LatticeCoeffs=[0.2 0.4]  denIgnore=on  FiltPerSampPopup=One filter per frame  IC=0  ICnum=0  ICden=0  roundingMode=Floor  overflowMode=off  ScaleValues=1  scaleValueFracLength=14  stageInFracLength=15  stageOutFracLength=15
  H2 : dsparch4/Digital Filter  DialogController=dspDDGCreate  DialogControllerArgs=DataTag17  TypePopup=IIR (poles & zeros)  IIRFiltStruct=Direct form II transposed  AllPoleFiltStruct=Direct form  FIRFiltStruct=Direct form  CoeffSource=Specify via dialog  NumCoeffs=[1 2]  DenCoeffs=[1 0.1]  BiQuadCoeffs=[1 0.3 0.4 1 0.1 0.2]  LatticeCoeffs=[0.2 0.4]  denIgnore=on  FiltPerSampPopup=One filter per frame  IC=0  ICnum=0  ICden=0  roundingMode=Floor  overflowMode=off  ScaleValues=1  scaleValueFracLength=14  stageInFracLength=15  stageOutFracLength=15
  H3 : dsparch4/Digital Filter  DialogController=dspDDGCreate  DialogControllerArgs=DataTag18  TypePopup=IIR (poles & zeros)  IIRFiltStruct=Direct form II transposed  AllPoleFiltStruct=Direct form  FIRFiltStruct=Direct form  CoeffSource=Specify via dialog  NumCoeffs=[1 2]  DenCoeffs=[1 0.1]  BiQuadCoeffs=[1 0.3 0.4 1 0.1 0.2]  LatticeCoeffs=[0.2 0.4]  denIgnore=on  FiltPerSampPopup=One filter per frame  IC=0  ICnum=0  ICden=0  roundingMode=Floor  overflowMode=off  ScaleValues=1  scaleValueFracLength=14  stageInFracLength=15  stageOutFracLength=15
  H4 : dsparch4/Digital Filter  DialogController=dspDDGCreate  DialogControllerArgs=DataTag19  TypePopup=IIR (poles & zeros)  IIRFiltStruct=Direct form II transposed  AllPoleFiltStruct=Direct form  FIRFiltStruct=Direct form  CoeffSource=Specify via dialog  NumCoeffs=[1 2]  DenCoeffs=[1 0.1]  BiQuadCoeffs=[1 0.3 0.4 1 0.1 0.2]  LatticeCoeffs=[0.2 0.4]  denIgnore=on  FiltPerSampPopup=One filter per frame  IC=0  ICnum=0  ICden=0  roundingMode=Floor  overflowMode=off  ScaleValues=1  scaleValueFracLength=14  stageInFracLength=15  stageOutFracLength=15
  SW : cdsSwitch1/Subsystem
  Sum{,1..7} (8 alike) : Sum  Inputs=|++
  V1 : dsparch4/Digital Filter  DialogController=dspDDGCreate  DialogControllerArgs=DataTag20  TypePopup=IIR (poles & zeros)  IIRFiltStruct=Direct form II transposed  AllPoleFiltStruct=Direct form  FIRFiltStruct=Direct form  CoeffSource=Specify via dialog  NumCoeffs=[1 2]  DenCoeffs=[1 0.1]  BiQuadCoeffs=[1 0.3 0.4 1 0.1 0.2]  LatticeCoeffs=[0.2 0.4]  denIgnore=on  FiltPerSampPopup=One filter per frame  IC=0  ICnum=0  ICden=0  roundingMode=Floor  overflowMode=off  ScaleValues=1  scaleValueFracLength=14  stageInFracLength=15  stageOutFracLength=15
  V2 : dsparch4/Digital Filter  DialogController=dspDDGCreate  DialogControllerArgs=DataTag21  TypePopup=IIR (poles & zeros)  IIRFiltStruct=Direct form II transposed  AllPoleFiltStruct=Direct form  FIRFiltStruct=Direct form  CoeffSource=Specify via dialog  NumCoeffs=[1 2]  DenCoeffs=[1 0.1]  BiQuadCoeffs=[1 0.3 0.4 1 0.1 0.2]  LatticeCoeffs=[0.2 0.4]  denIgnore=on  FiltPerSampPopup=One filter per frame  IC=0  ICnum=0  ICden=0  roundingMode=Floor  overflowMode=off  ScaleValues=1  scaleValueFracLength=14  stageInFracLength=15  stageOutFracLength=15
  V3 : dsparch4/Digital Filter  DialogController=dspDDGCreate  DialogControllerArgs=DataTag22  TypePopup=IIR (poles & zeros)  IIRFiltStruct=Direct form II transposed  AllPoleFiltStruct=Direct form  FIRFiltStruct=Direct form  CoeffSource=Specify via dialog  NumCoeffs=[1 2]  DenCoeffs=[1 0.1]  BiQuadCoeffs=[1 0.3 0.4 1 0.1 0.2]  LatticeCoeffs=[0.2 0.4]  denIgnore=on  FiltPerSampPopup=One filter per frame  IC=0  ICnum=0  ICden=0  roundingMode=Floor  overflowMode=off  ScaleValues=1  scaleValueFracLength=14  stageInFracLength=15  stageOutFracLength=15
  V4 : dsparch4/Digital Filter  DialogController=dspDDGCreate  DialogControllerArgs=DataTag23  TypePopup=IIR (poles & zeros)  IIRFiltStruct=Direct form II transposed  AllPoleFiltStruct=Direct form  FIRFiltStruct=Direct form  CoeffSource=Specify via dialog  NumCoeffs=[1 2]  DenCoeffs=[1 0.1]  BiQuadCoeffs=[1 0.3 0.4 1 0.1 0.2]  LatticeCoeffs=[0.2 0.4]  denIgnore=on  FiltPerSampPopup=One filter per frame  IC=0  ICnum=0  ICden=0  roundingMode=Floor  overflowMode=off  ScaleValues=1  scaleValueFracLength=14  stageInFracLength=15  stageOutFracLength=15
  OutV1 : Outport
  OutV2 : Outport  Port=2
  OutV3 : Outport  Port=3
  OutV4 : Outport  Port=4
  OutH1 : Outport  Port=5
  OutH2 : Outport  Port=6
  OutH3 : Outport  Port=7
  OutH4 : Outport  Port=8
  wires:
  GAIN/1 -> SW/1
  GAIN/2 -> SW/2
  GAIN/3 -> SW/3
  GAIN/4 -> SW/4
  GAIN/5 -> SW/5
  GAIN/6 -> SW/6
  GAIN/7 -> SW/7
  GAIN/8 -> SW/8
  V1DC/1 -> Sum/2
  V2DC/1 -> Sum1/2
  V3DC/1 -> Sum2/2
  V4DC/1 -> Sum3/2
  H1DC/1 -> Sum4/2
  H2DC/1 -> Sum5/2
  H3DC/1 -> Sum6/2
  H4DC/1 -> Sum7/2
  Sum4/1 -> H1/1
  Sum5/1 -> H2/1
  Sum6/1 -> H3/1
  Sum7/1 -> H4/1
  Sum3/1 -> V4/1
  Sum2/1 -> V3/1
  Sum1/1 -> V2/1
  Sum/1 -> V1/1
  V1In/1 -> Sum/1
  V2In/1 -> Sum1/1
  V3In/1 -> Sum2/1
  V4In/1 -> Sum3/1
  H1In/1 -> Sum4/1
  H2In/1 -> Sum5/1
  H3In/1 -> Sum6/1
  H4In/1 -> Sum7/1
  V1/1 -> GAIN/1
  V2/1 -> GAIN/2
  V3/1 -> GAIN/3
  V4/1 -> GAIN/4
  H1/1 -> GAIN/5
  H2/1 -> GAIN/6
  H3/1 -> GAIN/7
  H4/1 -> GAIN/8
  SW/1 -> OutV1/1
  SW/2 -> OutV2/1
  SW/3 -> OutV3/1
  SW/4 -> OutV4/1
  SW/5 -> OutH1/1
  SW/6 -> OutH2/1
  SW/7 -> OutH3/1
  SW/8 -> OutH4/1

== system sei/BSC_DC_BIAS ==
  {1..6} (6 alike) : cdsEpicsIn/Subsystem
  MTRX : Matrix8x/Subsystem
  SW : cdsSwitch1/Subsystem
  V1 : Outport
  V2 : Outport  Port=2
  V3 : Outport  Port=3
  V4 : Outport  Port=4
  H1 : Outport  Port=5
  H2 : Outport  Port=6
  H3 : Outport  Port=7
  H4 : Outport  Port=8
  wires:
  1/1 -> MTRX/1
  2/1 -> MTRX/2
  3/1 -> MTRX/3
  4/1 -> MTRX/4
  5/1 -> MTRX/5
  6/1 -> MTRX/6
  MTRX/1 -> SW/1
  MTRX/2 -> SW/2
  MTRX/3 -> SW/3
  MTRX/4 -> SW/4
  MTRX/5 -> SW/5
  MTRX/6 -> SW/6
  MTRX/7 -> SW/7
  MTRX/8 -> SW/8
  SW/1 -> V1/1
  SW/2 -> V2/1
  SW/3 -> V3/1
  SW/4 -> V4/1
  SW/5 -> H1/1
  SW/6 -> H2/1
  SW/7 -> H3/1
  SW/8 -> H4/1

== system sei/BSC_FIR ==
  X1 : Inport  Port=1  LatchInput=off
  Y1 : Inport  Port=2  LatchInput=off
  X2 : Inport  Port=3  LatchInput=off
  Y2 : Inport  Port=4  LatchInput=off
  MTRX : Matrix88/Subsystem
  X_OUT : dsparch4/Digital Filter  DialogController=dspDDGCreate  DialogControllerArgs=DataTag24  TypePopup=IIR (poles & zeros)  IIRFiltStruct=Direct form II transposed  AllPoleFiltStruct=Direct form  FIRFiltStruct=Direct form  CoeffSource=Specify via dialog  NumCoeffs=[1 2]  DenCoeffs=[1 0.1]  BiQuadCoeffs=[1 0.3 0.4 1 0.1 0.2]  LatticeCoeffs=[0.2 0.4]  denIgnore=on  FiltPerSampPopup=One filter per frame  IC=0  ICnum=0  ICden=0  roundingMode=Floor  overflowMode=off  ScaleValues=1  scaleValueFracLength=14  stageInFracLength=15  stageOutFracLength=15
  Y_OUT : dsparch4/Digital Filter  DialogController=dspDDGCreate  DialogControllerArgs=DataTag25  TypePopup=IIR (poles & zeros)  IIRFiltStruct=Direct form II transposed  AllPoleFiltStruct=Direct form  FIRFiltStruct=Direct form  CoeffSource=Specify via dialog  NumCoeffs=[1 2]  DenCoeffs=[1 0.1]  BiQuadCoeffs=[1 0.3 0.4 1 0.1 0.2]  LatticeCoeffs=[0.2 0.4]  denIgnore=on  FiltPerSampPopup=One filter per frame  IC=0  ICnum=0  ICden=0  roundingMode=Floor  overflowMode=off  ScaleValues=1  scaleValueFracLength=14  stageInFracLength=15  stageOutFracLength=15
  X : Outport
  Y : Outport  Port=2
  wires:
  MTRX/1 -> X_OUT/1
  MTRX/2 -> Y_OUT/1
  X1/1 -> MTRX/1
  X_OUT/1 -> X/1
  Y1/1 -> MTRX/2
  X2/1 -> MTRX/3
  Y2/1 -> MTRX/4
  Y_OUT/1 -> Y/1
